simulink model "ex3_sim1"  (R2019b)
settings: Solver=ode45  StartTime=0.0  StopTime=2  MaxStep=0.01  RelTol=1e-3
undefined symbols (not defined in the file): Ad, Ar, denC, denH, denP, denQ, denW, km, numC, numH, numP, numQ, numW, rads2rpm, t0d, t0r, Ts
Description:
  | Riccardo Antonello (riccardo.antonello@unipd.it)
  | 
  | June 18, 2020
  | 
  | Dept. of Information Engineering, University of Padova
settings Model: Creator=riccardo  LastModifiedBy=riccardo
settings DataIOCC: ReturnWorkspaceOutputs=off
settings DebuggingCC: ArithmeticOperatorsInVariantConditions=warning
settings SFSimCC: CustomCodeUndefinedFunction=UseInterfaceOnly

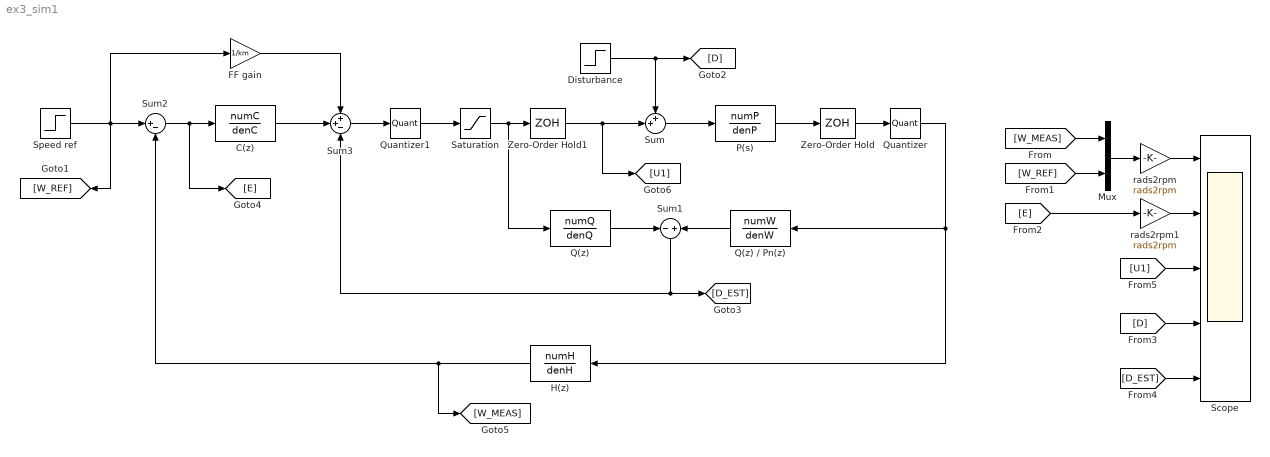
== system ex3_sim1 ==
  C(z) : DiscreteTransferFcn  Numerator=numC  Denominator=denC  SampleTime=Ts
  Disturbance : Step  Time=t0d  After=Ad  SampleTime=0
  FF gain : Gain  Gain=1/km
  H(z) : DiscreteTransferFcn  Numerator=numH  Denominator=denH  SampleTime=Ts
  Mux : Mux  Inputs=2
  P(s) : TransferFcn  Numerator=numP  Denominator=denP
  Q(z) : DiscreteTransferFcn  Numerator=numQ  Denominator=denQ  SampleTime=Ts
  Q(z) / Pn(z) : DiscreteTransferFcn  Numerator=numW  Denominator=denW  SampleTime=Ts
  Quantizer : Quantizer  QuantizationInterval=2*pi/2000
  Quantizer1 : Quantizer  QuantizationInterval=20/2^10
  Saturation : Saturate  UpperLimit=10  LowerLimit=-10
  Scope : Scope  NumInputPorts=5
  Speed ref : Step  Time=t0r  After=Ar  SampleTime=Ts
  Sum : Sum  Inputs=++|
  Sum1 : Sum  Inputs=-+
  Sum2 : Sum  Inputs=|+-
  Sum3 : Sum  Inputs=++-
  Zero-Order Hold : ZeroOrderHold  SampleTime=Ts
  Zero-Order Hold1 : ZeroOrderHold  SampleTime=Ts
  rads2rpm : Gain  Gain=rads2rpm
  rads2rpm1 : Gain  Gain=rads2rpm
  wires:
  Sum/1 -> P(s)/1
  P(s)/1 -> Zero-Order Hold/1
  Q(z)/1 -> Sum1/1
  Q(z) / Pn(z)/1 -> Sum1/2
  Saturation/1 -> Q(z)/1, Zero-Order Hold1/1
  Sum2/1 -> [E], C(z)/1
  Speed ref/1 -> FF gain/1, Sum2/1, [W_REF]
  Sum3/1 -> Quantizer1/1
  Mux/1 -> rads2rpm/1
  [W_MEAS] -> Mux/1
  [W_REF] -> Mux/2
  [E] -> rads2rpm1/1
  rads2rpm/1 -> Scope/1
  Sum1/1 -> [D_EST], Sum3/3
  Disturbance/1 -> [D], Sum/1
  Zero-Order Hold/1 -> Quantizer/1
  Quantizer/1 -> Q(z) / Pn(z)/1, H(z)/1
  Zero-Order Hold1/1 -> [U1], Sum/2
  Quantizer1/1 -> Saturation/1
  rads2rpm1/1 -> Scope/2
  H(z)/1 -> [W_MEAS], Sum2/2
  C(z)/1 -> Sum3/2
  FF gain/1 -> Sum3/1
  [D_EST] -> Scope/5
  [D] -> Scope/4
  [U1] -> Scope/3
